simulink model "harmonic_osc"  (R2022a)
settings: Solver=VariableStepAuto  StartTime=0.0  StopTime=100  RelTol=1e-3
settings Model: Creator=Home computer  LastModifiedBy=Home computer

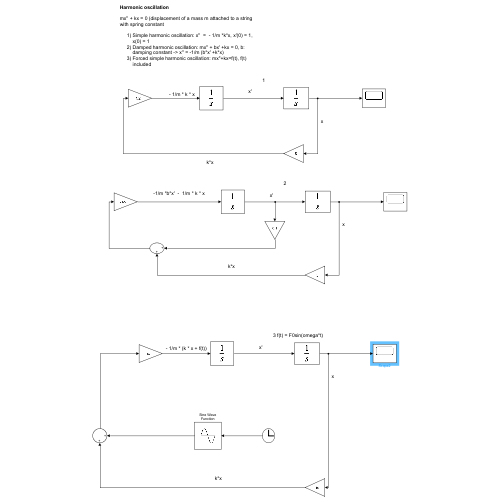
[thumbnail: Simulink's stored preview of the top-level diagram]
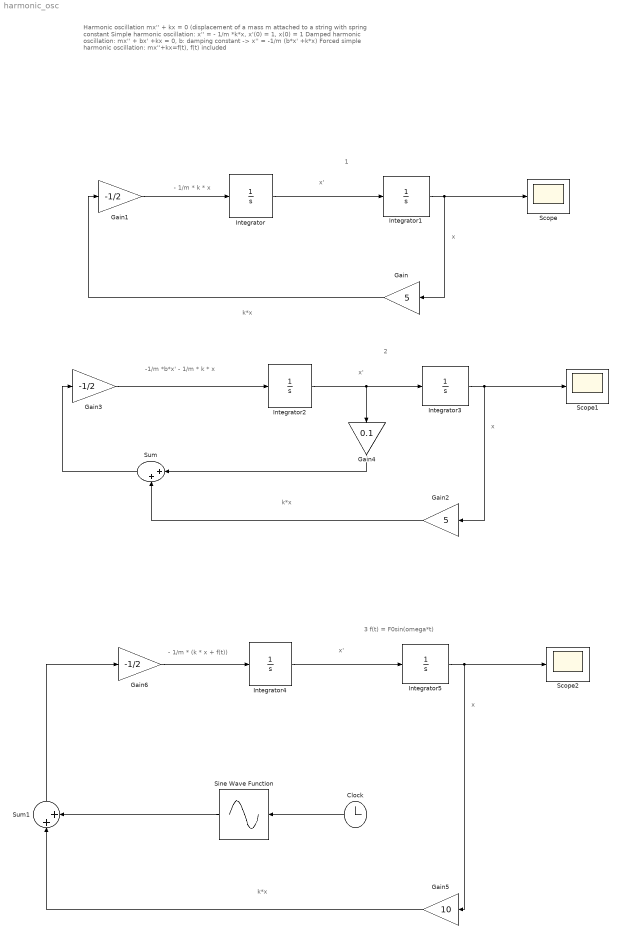
== system harmonic_osc ==
  note: 1
  note: - 1/m * k * x
  note: k*x
  note: x
  note: x'
  note: Harmonic oscillation
      |
      | mx'' + kx = 0 (displacement of a mass m attached to a string with spring constant
      |
      | Simple harmonic oscillation: x'' = - 1/m *k*x, x'(0) = 1, x(0) = 1
      | Damped harmonic oscillation: mx'' + bx' +kx = 0, b: damping constant -> x'' = -1/m (b*x' +k*x)
      | Forced simple harmonic oscillation: mx''+kx=f(t), f(t) included
  note: x'
  note: -1/m *b*x' - 1/m * k * x
  note: k*x
  note: 2
  note: x
  note: x'
  note: - 1/m * (k * x + f(t))
  note: k*x
  note: 3 f(t) = F0sin(omega*t)
  note: x
  Clock : Clock
  Gain : Gain  Gain=5
  Gain1 : Gain  Gain=-1/2
  Gain2 : Gain  Gain=5
  Gain3 : Gain  Gain=-1/2
  Gain4 : Gain  Gain=0.1
  Gain5 : Gain  Gain=10
  Gain6 : Gain  Gain=-1/2
  Integrator{,1..5} (6 alike) : Integrator  InitialCondition=1
  Scope : Scope
  Scope1 : Scope
  Scope2 : Scope
  Sine Wave Function : Sin  TimeSource=Use external signal  Frequency=2  SampleTime=0
  Sum : Sum  Inputs=|++
  Sum1 : Sum  Inputs=|++
  wires:
  Integrator/1 -> Integrator1/1
  Integrator1/1 -> Scope/1, Gain/1
  Gain/1 -> Gain1/1
  Gain1/1 -> Integrator/1
  Gain3/1 -> Integrator2/1
  Gain2/1 -> Sum/2
  Integrator3/1 -> Scope1/1, Gain2/1
  Integrator2/1 -> Gain4/1, Integrator3/1
  Gain4/1 -> Sum/1
  Sum/1 -> Gain3/1
  Gain6/1 -> Integrator4/1
  Gain5/1 -> Sum1/1
  Integrator5/1 -> Scope2/1, Gain5/1
  Integrator4/1 -> Integrator5/1
  Clock/1 -> Sine Wave Function/1
  Sine Wave Function/1 -> Sum1/2
  Sum1/1 -> Gain6/1
